simulink model "UAV01_step2"  (R2025a)
settings: Solver=VariableStepAuto  StartTime=0.0  StopTime=10.0  RelTol=1e-3
settings Model: Creator=ayeo  LastModifiedBy=ayeo

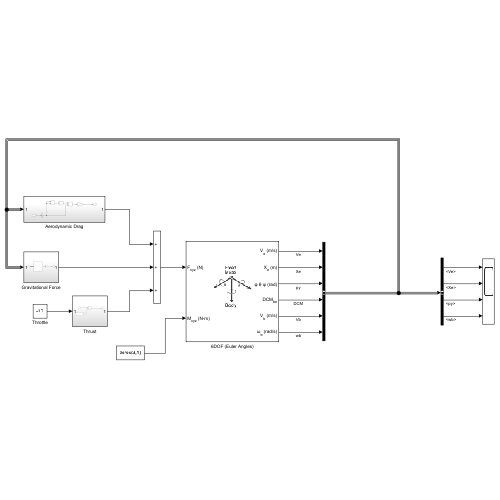
[thumbnail: Simulink's stored preview of the top-level diagram]
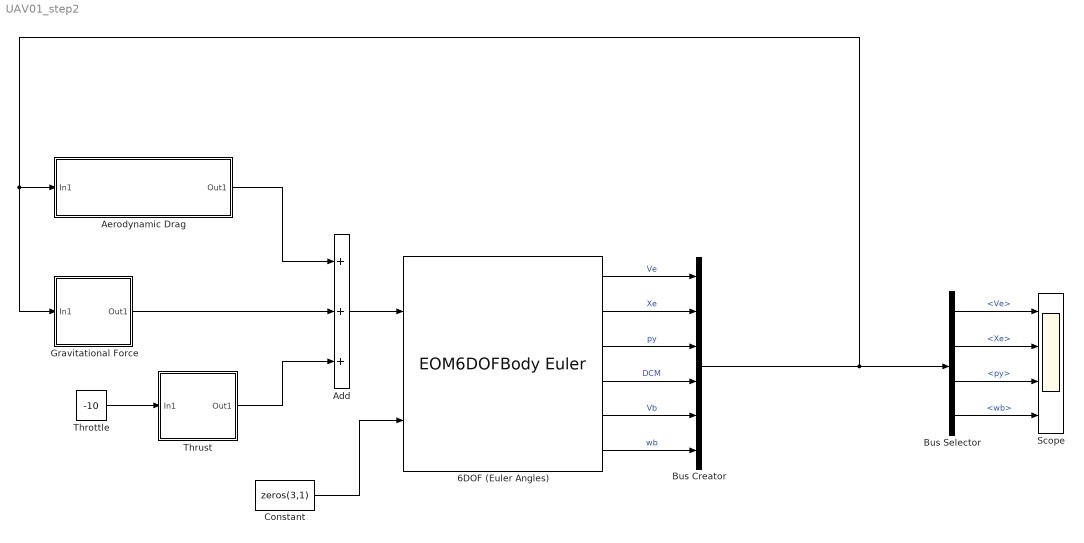
== system UAV01_step2 ==
  6DOF (Euler Angles) : EOM6DOFBodyEuler
  Add : Sum  Inputs=+++
  Aerodynamic Drag : Subsystem
  Bus Creator : BusCreator  Inputs=6
  Bus Selector : BusSelector  OutputSignals=Ve,Xe,py,wb
  Constant : Constant  Value=zeros(3,1)
  Gravitational Force : Subsystem
  Scope : Scope  NumInputPorts=4
      settings: ActiveDisplayYMinimum=-2.072289387003964  ActiveDisplayYMaximum=0.23025437633377374
  Throttle : Constant  Value=-10
  Thrust : Subsystem
  wires:
  Constant/1 -> 6DOF (Euler Angles)/2
  6DOF (Euler Angles)/1 -> Bus Creator/1  "Ve"
  6DOF (Euler Angles)/3 -> Bus Creator/3  "py"
  6DOF (Euler Angles)/2 -> Bus Creator/2  "Xe"
  6DOF (Euler Angles)/4 -> Bus Creator/4  "DCM"
  6DOF (Euler Angles)/5 -> Bus Creator/5  "Vb"
  6DOF (Euler Angles)/6 -> Bus Creator/6  "wb"
  Bus Creator/1 -> Aerodynamic Drag/1(In1), Gravitational Force/1(In1), Bus Selector/1
  Bus Selector/1 -> Scope/1  "<Ve>"
  Bus Selector/2 -> Scope/2  "<Xe>"
  Bus Selector/3 -> Scope/3  "<py>"
  Bus Selector/4 -> Scope/4  "<wb>"
  Add/1 -> 6DOF (Euler Angles)/1
  Throttle/1 -> Thrust/1(In1)
  Thrust/1(Out1) -> Add/3
  Gravitational Force/1(Out1) -> Add/2
  Aerodynamic Drag/1(Out1) -> Add/1

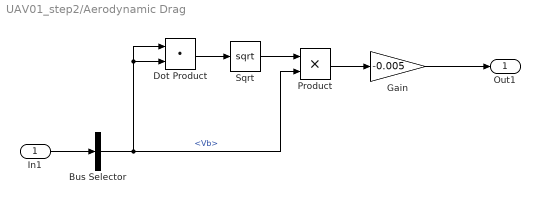
== system UAV01_step2/Aerodynamic Drag ==
  In1 : Inport
  Bus Selector : BusSelector  OutputSignals=Vb
  Dot Product : DotProduct  OutDataTypeStr=Inherit: Inherit via internal rule
  Gain : Gain  Gain=-0.005
  Product : Product
  Sqrt : Sqrt
  Out1 : Outport
  wires:
  In1/1 -> Bus Selector/1
  Bus Selector/1 -> Product/2, Dot Product/2, Dot Product/1  "<Vb>"
  Dot Product/1 -> Sqrt/1
  Sqrt/1 -> Product/1
  Product/1 -> Gain/1
  Gain/1 -> Out1/1

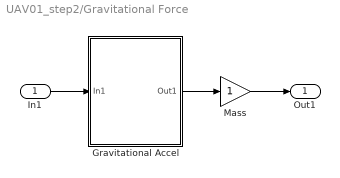
== system UAV01_step2/Gravitational Force ==
  In1 : Inport
  Gravitational Accel : Subsystem
  Mass : Gain
  Out1 : Outport
  wires:
  Gravitational Accel/1(Out1) -> Mass/1
  In1/1 -> Gravitational Accel/1(In1)
  Mass/1 -> Out1/1

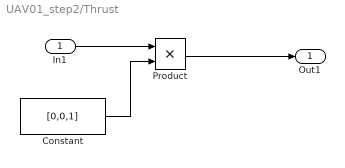
== system UAV01_step2/Thrust ==
  In1 : Inport
  Constant : Constant  Value=[0,0,1]
  Product : Product
  Out1 : Outport
  wires:
  In1/1 -> Product/1
  Constant/1 -> Product/2
  Product/1 -> Out1/1

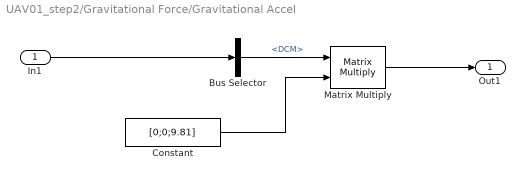
== system UAV01_step2/Gravitational Force/Gravitational Accel ==
  In1 : Inport
  Bus Selector : BusSelector  OutputSignals=DCM
  Constant : Constant  Value=[0;0;9.81]
  Matrix Multiply : Product  Multiplication=Matrix(*)
  Out1 : Outport
  wires:
  In1/1 -> Bus Selector/1
  Bus Selector/1 -> Matrix Multiply/1  "<DCM>"
  Constant/1 -> Matrix Multiply/2
  Matrix Multiply/1 -> Out1/1
